simulink model "dz_1_simul_model"  (R2026a)
settings: Solver=VariableStepAuto  StopTime=30
values from neighbouring files (symbols this model uses):
  g = 9.81    [dz_1_model.m]
  mass_quadrotor = 1.07    [dz_1_model.m]
settings Model: Creator=vas77  LastModifiedBy=vas77
settings HardwareCC: ProdHWDeviceType=AMD->x86-64 (Windows64)
settings RTWCC: BuildConfiguration=Faster Runs

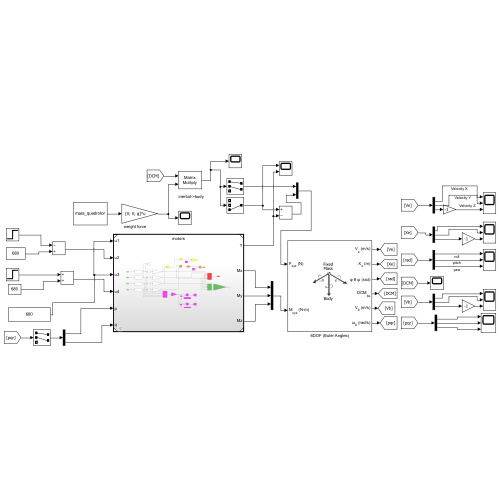
[thumbnail: Simulink's stored preview of the top-level diagram]
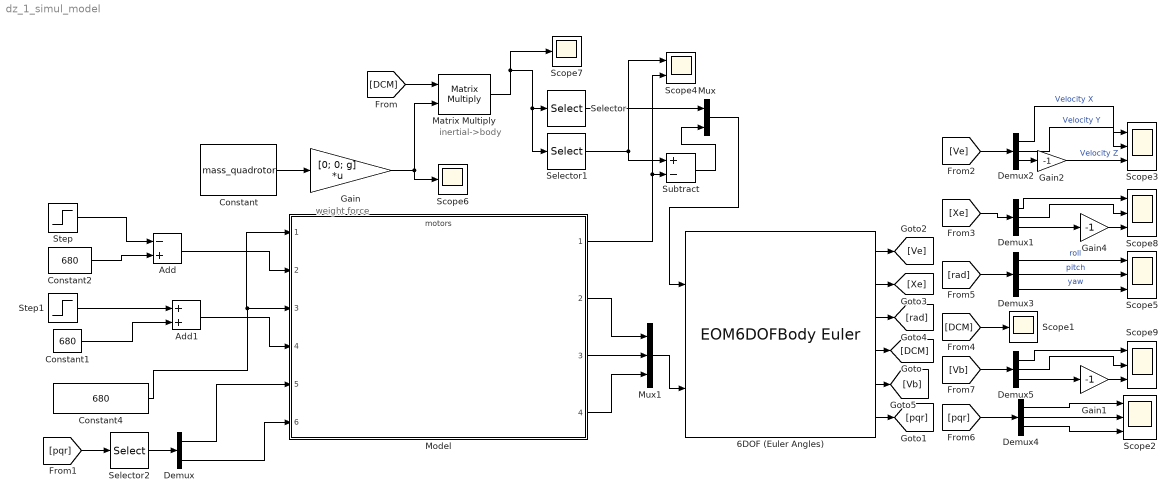
== system dz_1_simul_model ==
  note: weight force
  note: inertial->body
  6DOF (Euler Angles) : EOM6DOFBodyEuler  mass_0=mass_quadrotor  inertia=I
  Add : Sum  Inputs=-+
  Add1 : Sum
  Constant : Constant  Value=mass_quadrotor  VectorParams1D=off
  Constant1 : Constant  Value=680
  Constant2 : Constant  Value=680
  Constant4 : Constant  Value=680
  Demux : Demux  Outputs=2
  Demux{1..5} (5 alike) : Demux  Outputs=3
  Gain : Gain  Gain=[0; 0; g]  Multiplication=Matrix(K*u)
  Gain1 : Gain  Gain=-1
  Gain2 : Gain  Gain=-1
  Gain4 : Gain  Gain=-1
  Matrix Multiply : Product  Multiplication=Matrix(*)
  Model : ModelReference  ModelNameDialog=motors.slx  SimulationMode=Normal  ModelReferenceVersion=1.19
  Mux : Mux  Inputs=2
  Mux1 : Mux  Inputs=3
  Scope1 : Scope
      settings: ActiveDisplayYMinimum=-1.2499491050427127  ActiveDisplayYMaximum=1.2499943450047457
  Scope{2..3,5,8..9} (5 alike) : Scope  NumInputPorts=3
      Scope2 settings: ActiveDisplayYMinimum=-1  ActiveDisplayYMaximum=1  DataLoggingVariableName=ScopeData2
      Scope3 settings: Title=Velocity ( Earth )  ActiveDisplayYMinimum=-11.464025219833569  ActiveDisplayYMaximum=93.3199733053954  YLabel=Speed(m/s)
      Scope5 settings: Title=Roll, pitch, yaw  ActiveDisplayYMinimum=-3.9033370990477581  ActiveDisplayYMaximum=3.3841334226447608  YLabel=Roll, pitch, yaw( rad )  DataLoggingVariableName=ScopeData3
      Scope8 settings: ActiveDisplayString=3  Title=Displacement Z (m)  ActiveDisplayYMinimum=-161.26863397971496  ActiveDisplayYMaximum=1447.5005395724611  YLabel=Displacement Z (m)  DataLoggingVariableName=ScopeData8
      Scope9 settings: ActiveDisplayString=3  Title=Velocity Z  ActiveDisplayYMinimum=-186.94116082031456  ActiveDisplayYMaximum=119.00417486295329  YLabel=Speed(m/s)  DataLoggingVariableName=ScopeData5
  Scope4 : Scope  NumInputPorts=2
      settings: ActiveDisplayYMinimum=5.9584764482034869  ActiveDisplayYMaximum=15.675635410083268  DataLoggingVariableName=ScopeData4
  Scope6 : Scope
      settings: ActiveDisplayYMinimum=5.1775949245841977  ActiveDisplayYMaximum=10.902189225640303  DataLoggingVariableName=ScopeData6
  Scope7 : Scope
      settings: ActiveDisplayYMinimum=-1  ActiveDisplayYMaximum=1  DataLoggingVariableName=ScopeData7
  Selector : Selector  IndexMode=Zero-based  InputPortWidth=3  IndexOptions=Index vector (dialog)  Indices=[0 1]  OutputSizes=1
  Selector1 : Selector  IndexMode=Zero-based  InputPortWidth=3  IndexOptions=Index vector (dialog)  Indices=[2]  OutputSizes=1
  Selector2 : Selector  IndexMode=Zero-based  InputPortWidth=3  IndexOptions=Index vector (dialog)  Indices=[0 1]  OutputSizes=1
  Step : Step  Time=4  FinalValue=10  SampleTime=0
  Step1 : Step  Time=4  FinalValue=10  SampleTime=0
  Subtract : Sum  Inputs=+-
  wires:
  Constant/1 -> Gain/1
  [DCM] -> Matrix Multiply/1
  Gain/1 -> Matrix Multiply/2, Scope6/1
  Matrix Multiply/1 -> Scope7/1, Selector1/1, Selector/1
  Selector1/1 -> Scope4/1, Subtract/1
  Subtract/1 -> Mux/2
  Selector/1 -> Mux/1
  Model/1 -> Scope4/2, Subtract/2
  Mux/1 -> 6DOF (Euler Angles)/1
  Model/2 -> Mux1/1
  Model/3 -> Mux1/2
  Model/4 -> Mux1/3
  Mux1/1 -> 6DOF (Euler Angles)/2
  6DOF (Euler Angles)/4 -> [DCM]
  [pqr] -> Selector2/1
  Demux/1 -> Model/5
  Demux/2 -> Model/6
  Selector2/1 -> Demux/1
  6DOF (Euler Angles)/2 -> [Xe]
  Demux1/1 -> Scope8/1
  Demux1/2 -> Scope8/2
  Demux1/3 -> Gain4/1
  Gain4/1 -> Scope8/3
  6DOF (Euler Angles)/1 -> [Ve]
  Demux2/3 -> Gain2/1
  Gain2/1 -> Scope3/3  "Velocity Z"
  Demux2/2 -> Scope3/2  "Velocity Y"
  Demux2/1 -> Scope3/1  "Velocity X"
  [DCM] -> Scope1/1
  [rad] -> Demux3/1
  Demux3/2 -> Scope5/2  "pitch"
  Demux3/1 -> Scope5/1  "roll"
  6DOF (Euler Angles)/3 -> [rad]
  6DOF (Euler Angles)/6 -> [pqr]
  Demux3/3 -> Scope5/3  "yaw"
  [pqr] -> Demux4/1
  Demux4/2 -> Scope2/2
  Demux4/3 -> Scope2/3
  Demux4/1 -> Scope2/1
  [Ve] -> Demux2/1
  [Xe] -> Demux1/1
  [Vb] -> Demux5/1
  Demux5/1 -> Scope9/1
  Demux5/2 -> Scope9/2
  Gain1/1 -> Scope9/3
  Demux5/3 -> Gain1/1
  6DOF (Euler Angles)/5 -> [Vb]
  Step/1 -> Add/1
  Constant2/1 -> Add/2
  Constant1/1 -> Add1/2
  Step1/1 -> Add1/1
  Constant4/1 -> Model/3, Model/1
  Add/1 -> Model/2
  Add1/1 -> Model/4
